simulink library "ams"  (Simulink 8.1)
settings: Solver=ode1  StartTime=0.0  StopTime=Inf  FixedStep=0.001  RelTol=1e-3
PostLoadFcn:
  | , if any(exist('dsrtsu_mdlpostloadfcn', 'file') == [2, 3, 6]), try dsrtsu_mdlpostloadfcn('Execute', bdroot); catch fprintf('Error in PostLoadFcn (dsrtsu_mdlpostloadfcn) for model "%s":\n %s\n', bdroot, lasterr); end, end,
undefined symbols (not defined in the file or in its folder): KIFO_AEBExistProbLimit_num, ZERO_INT
settings Model: DSRTSU_INTERNAL_RTI_VER=450  DSRTSU_INTERNAL_RTI_TYPE=rti1401  RTICANMMDATA=struct('GeneralSetupData',struct('modelroot','D:\ELN150201_TAIWAN\trunk\AdasDragon\software\sw_development\arch\app\ifo','generalsettings',struct('filesettings',struct('destfolder',struct('Name','RTICANMM_FILES','Check',1),'buildfolder',struct('Name','.','Check',1),'AbsDestfolder',struct('Name','D:\ELN150201_TAIWAN\trunk\AdasDragon\software\sw_development\arch\app\ifo\RTICANMM_FILES'),'AbsBuildfolder',struct('Name','D:\ELN150201_TAIWAN\trunk\AdasDragon\software\sw_development\arch\app\ifo'))),'options',struct('addpaths',1,'rmpaths',1,'addtrcexclusion',logical(1),'cannavigator',struct('checkmonitoring',0),'show_usrtrc',0,'use_usrtrc',0),'advanced',struct('options',[1 1 1 1 1 1 1 1 1 1 1 1 1 1 1 1 1 1 1 1 1 1 1 1 1 1 1 1 1 1 1 1 1 1 1 1 1 1 1 1 1 1 1 1 1 1 1 1 1 1 1 1 1 1 1 1 1 1 1 1 1 1 1 1 1 1 1 1 1 1 1 1 1 1 1 1 1 1 1 1 1 1 1 1 1 1 1 1 1 1 1 1 1 1 1 1 1 1 1 1]),'MPSetup',{{}},'modelname','ams','block','ams'))  DSRTSU_INTERNAL_RTIFPGA=40  Creator=tescamilla  LastModifiedBy=AT015555

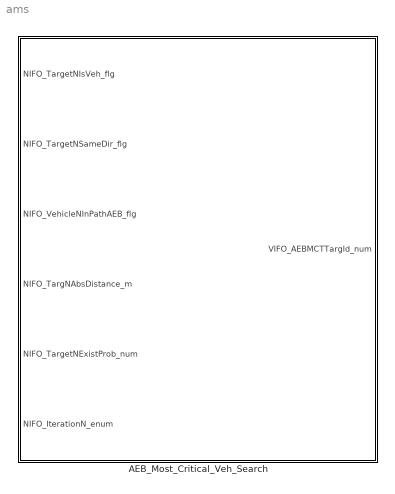
== system ams ==
  AEB_Most_Critical_Veh_Search : Subsystem

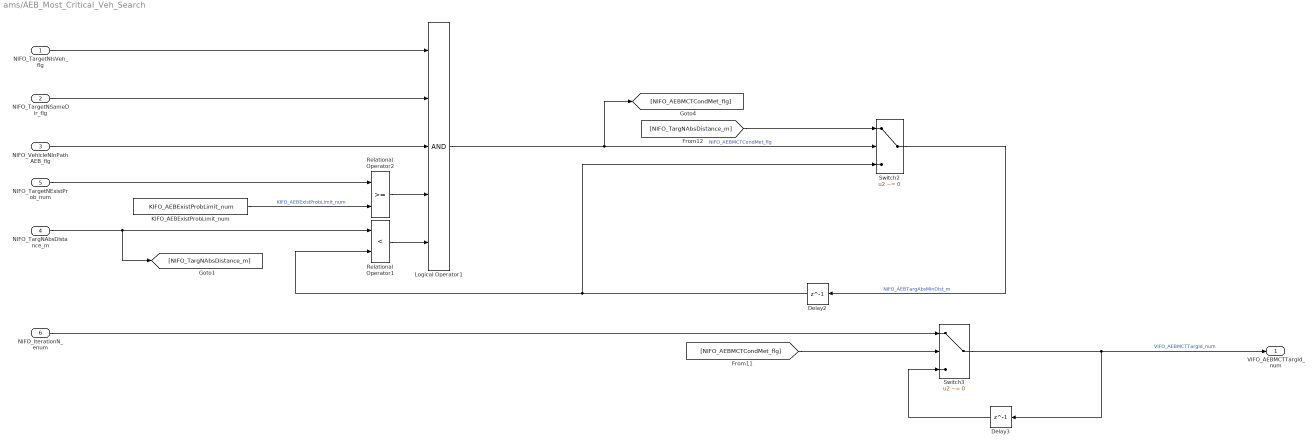
== system ams/AEB_Most_Critical_Veh_Search ==
  NIFO_TargetNIsVeh_flg : Inport
  NIFO_TargetNSameDir_flg : Inport  Port=2
  NIFO_VehicleNInPathAEB_flg : Inport  Port=3
  NIFO_TargNAbsDistance_m : Inport  Port=4
  NIFO_TargetNExistProb_num : Inport  Port=5
  NIFO_IterationN_enum : Inport  Port=6
  Delay2 : Delay  DelayLength=1  InitialCondition=1000
  Delay3 : Delay  DelayLength=1  InitialCondition=ZERO_INT
  KIFO_AEBExistProbLimit_num : Constant  Value=KIFO_AEBExistProbLimit_num
  Logical Operator1 : Logic  Inputs=5  AllPortsSameDT=off  OutDataTypeStr=boolean
  Relational Operator1 : RelationalOperator  Operator=<  OutDataTypeStr=boolean
  Relational Operator2 : RelationalOperator  OutDataTypeStr=boolean
  Switch2 : Switch  Criteria=u2 ~= 0
  Switch3 : Switch  Criteria=u2 ~= 0
  VIFO_AEBMCTTargId_num : Outport
  wires:
  Relational Operator2/1 -> Logical Operator1/4
  KIFO_AEBExistProbLimit_num/1 -> Relational Operator2/2  "KIFO_AEBExistProbLimit_num"
  NIFO_TargetNExistProb_num/1 -> Relational Operator2/1
  [NIFO_TargNAbsDistance_m] -> Switch2/1
  Logical Operator1/1 -> [NIFO_AEBMCTCondMet_flg], Switch2/2  "NIFO_AEBMCTCondMet_flg"
  Delay2/1 -> Switch2/3, Relational Operator1/2
  NIFO_IterationN_enum/1 -> Switch3/1
  Relational Operator1/1 -> Logical Operator1/5
  NIFO_TargNAbsDistance_m/1 -> [NIFO_TargNAbsDistance_m], Relational Operator1/1
  NIFO_TargetNIsVeh_flg/1 -> Logical Operator1/1
  [NIFO_AEBMCTCondMet_flg] -> Switch3/2
  NIFO_VehicleNInPathAEB_flg/1 -> Logical Operator1/3
  Switch3/1 -> Delay3/1, VIFO_AEBMCTTargId_num/1  "VIFO_AEBMCTTargId_num"
  Switch2/1 -> Delay2/1  "NIFO_AEBTargAbsMinDist_m"
  NIFO_TargetNSameDir_flg/1 -> Logical Operator1/2
  Delay3/1 -> Switch3/3
